simulink model "Motor_observer"  (R2019b)
settings: Solver=VariableStepAuto  StartTime=0.0  StopTime=10.0  RelTol=1e-3
undefined symbols (not defined in the file): c_m
libraries: simulink x1
settings Model: Creator=Олег  LastModifiedBy=Олег

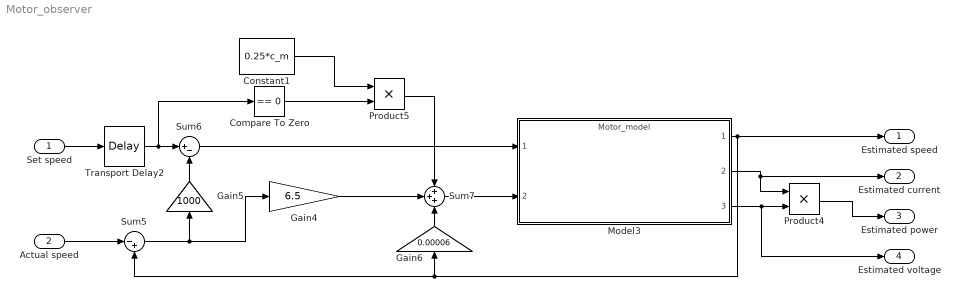
== system Motor_observer ==
  Set speed : Inport
  Actual speed : Inport  Port=2
  Compare To Zero : simulink/Logic and Bit Operations/Compare To Zero  relop===  OutDataTypeStr=uint8
  Constant1 : Constant  Value=0.25*c_m
  Gain4 : Gain  Gain=6.5
  Gain5 : Gain  Gain=1000
  Gain6 : Gain  Gain=0.00006
  Model3 : ModelReference  ModelNameDialog=Motor_model.slx  SimulationMode=Normal  ModelReferenceVersion=1.134
  Product4 : Product
  Product5 : Product
  Sum5 : Sum  Inputs=|-+
  Sum6 : Sum  Inputs=|+-
  Sum7 : Sum  Inputs=+++
  Transport Delay2 : TransportDelay  DelayTime=0.15
  Estimated speed : Outport
  Estimated current : Outport  Port=2
  Estimated power : Outport  Port=3
  Estimated voltage : Outport  Port=4
  wires:
  Sum7/1 -> Model3/2
  Gain6/1 -> Sum7/3
  Model3/2 -> Estimated current/1, Product4/1
  Product5/1 -> Sum7/1
  Gain5/1 -> Sum6/2
  Compare To Zero/1 -> Product5/2
  Actual speed/1 -> Sum5/1
  Product4/1 -> Estimated power/1
  Transport Delay2/1 -> Sum6/1, Compare To Zero/1
  Constant1/1 -> Product5/1
  Sum6/1 -> Model3/1
  Sum5/1 -> Gain4/1, Gain5/1
  Model3/3 -> Estimated voltage/1, Product4/2
  Model3/1 -> Estimated speed/1, Sum5/2, Gain6/1
  Gain4/1 -> Sum7/2
  Set speed/1 -> Transport Delay2/1
